simulink model "Sample11"  (R2021b)
settings: Solver=VariableStepAuto  StartTime=0.0  StopTime=10.0  RelTol=1e-3
settings Model: Creator=ygkwon  LastModifiedBy=ygkwon

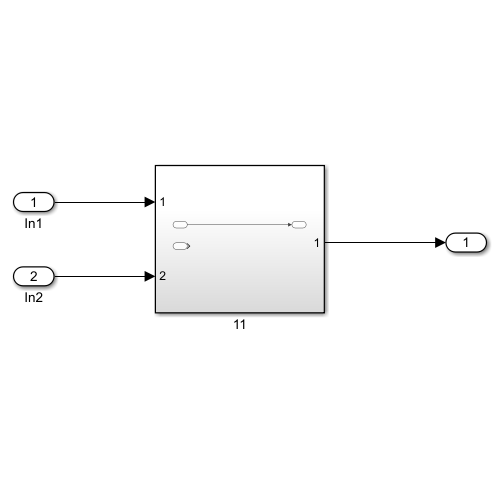
[thumbnail: Simulink's stored preview of the top-level diagram]
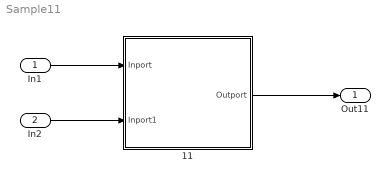
== system Sample11 ==
  In1 : Inport
  In2 : Inport  Port=2
  11 : Subsystem
  Out11 : Outport
  wires:
  In1/1 -> 11/1(Inport)
  In2/1 -> 11/2(Inport1)
  11/1(Outport) -> Out11/1

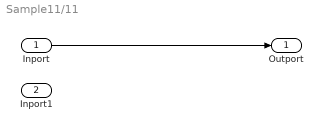
== system Sample11/11 ==
  Inport : Inport
  Inport1 : Inport  Port=2
  Outport : Outport
  wires:
  Inport/1 -> Outport/1
